simulink library "csc_prs_pressure_system_sim_lib"  (R2014b)
settings: Solver=ode45  StartTime=0.0  StopTime=10.0  RelTol=1e-3
undefined symbols (not defined in the file): egt_feed_pressure, gps_jump_seed, prs_10000psi_psi_to_counts_offset_cnv, prs_10000psi_psi_to_counts_slope_cnv, prs_1000psi_psi_to_counts_offset_cnv, prs_1000psi_psi_to_counts_slope_cnv, prs_500psi_psi_to_counts_offset_cnv, prs_500psi_psi_to_counts_slope_cnv, stm_time_step
libraries: util_common_lib x2, simulink x1, util_info_lib x1
settings Model: Creator=escrane  LastModifiedBy=mstewart

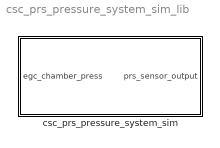
== system csc_prs_pressure_system_sim_lib ==
  csc_prs_pressure_system_sim : Subsystem  SystemSampleTime=stm_time_step

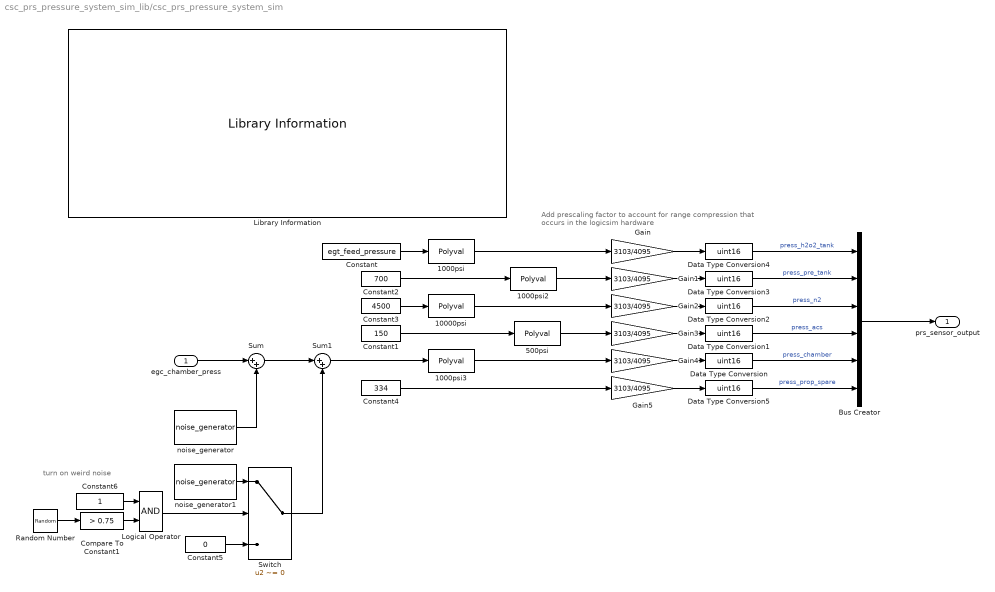
== system csc_prs_pressure_system_sim_lib/csc_prs_pressure_system_sim ==
  note: Add prescaling factor to account for range
      | compression that occurs in the logicsim hardware
  note: turn on weird noise
  egc_chamber_press : Inport
  10000psi : Polyval  Coefs=[prs_10000psi_psi_to_counts_slope_cnv prs_10000psi_psi_to_counts_offset_cnv]
  1000psi : Polyval  Coefs=[prs_1000psi_psi_to_counts_slope_cnv prs_1000psi_psi_to_counts_offset_cnv]
  1000psi2 : Polyval  Coefs=[prs_1000psi_psi_to_counts_slope_cnv prs_1000psi_psi_to_counts_offset_cnv]
  1000psi3 : Polyval  Coefs=[3.2975 823.8835]
  500psi : Polyval  Coefs=[prs_500psi_psi_to_counts_slope_cnv prs_500psi_psi_to_counts_offset_cnv]
  Bus Creator : BusCreator  Inputs=6
  Compare To Constant1 : simulink/Logic and Bit Operations/Compare To Constant  relop=>  const=0.75  OutDataTypeStr=boolean
  Constant : Constant  Value=egt_feed_pressure  OutDataTypeStr=double
  Constant1 : Constant  Value=150  OutDataTypeStr=double
  Constant2 : Constant  Value=700  OutDataTypeStr=double
  Constant3 : Constant  Value=4500  OutDataTypeStr=double
  Constant4 : Constant  Value=334  OutDataTypeStr=double
  Constant5 : Constant  Value=0  OutDataTypeStr=double
  Constant6 : Constant  OutDataTypeStr=double
  Data Type Conversion{,1..5} (6 alike) : DataTypeConversion  OutDataTypeStr=uint16
  Gain{,1..5} (6 alike) : Gain  Gain=3103/4095
  Library Information : util_info_lib/Library Information  owner='escrane'
  Logical Operator : Logic  AllPortsSameDT=off  OutDataTypeStr=boolean
  Random Number : RandomNumber  Seed=gps_jump_seed  SampleTime=0.01
  Sum : Sum  Inputs=|++
  Sum1 : Sum  Inputs=|++
  Switch : Switch  Criteria=u2 ~= 0
  noise_generator : util_common_lib/noise_generator  std_dev=2  bias=0  seed=89  on=1  sample_time=sim_time_step_size
  noise_generator1 : util_common_lib/noise_generator  std_dev=14  bias=0  seed=89  on=1  sample_time=sim_time_step_size
  prs_sensor_output : Outport
  wires:
  Constant6/1 -> Logical Operator/1
  Compare To Constant1/1 -> Logical Operator/2
  Switch/1 -> Sum1/2
  Sum/1 -> Sum1/1
  Constant5/1 -> Switch/3
  noise_generator1/1 -> Switch/1
  Logical Operator/1 -> Switch/2
  Random Number/1 -> Compare To Constant1/1
  Gain5/1 -> Data Type Conversion5/1
  Gain4/1 -> Data Type Conversion/1
  Gain3/1 -> Data Type Conversion1/1
  Gain2/1 -> Data Type Conversion2/1
  Gain1/1 -> Data Type Conversion3/1
  Gain/1 -> Data Type Conversion4/1
  1000psi3/1 -> Gain4/1
  Sum1/1 -> 1000psi3/1
  noise_generator/1 -> Sum/2
  egc_chamber_press/1 -> Sum/1
  Constant/1 -> 1000psi/1
  Data Type Conversion3/1 -> Bus Creator/2  "press_pre_tank"
  Data Type Conversion2/1 -> Bus Creator/3  "press_n2"
  Data Type Conversion1/1 -> Bus Creator/4  "press_acs"
  Data Type Conversion/1 -> Bus Creator/5  "press_chamber"
  Data Type Conversion5/1 -> Bus Creator/6  "press_prop_spare"
  Bus Creator/1 -> prs_sensor_output/1
  Data Type Conversion4/1 -> Bus Creator/1  "press_h2o2_tank"
  Constant2/1 -> 1000psi2/1
  Constant3/1 -> 10000psi/1
  Constant1/1 -> 500psi/1
  500psi/1 -> Gain3/1
  10000psi/1 -> Gain2/1
  1000psi2/1 -> Gain1/1
  1000psi/1 -> Gain/1
  Constant4/1 -> Gain5/1
